simulink model "sim_ukf_est_motor_3para"  (R2020b)
settings: Solver=ode1  StartTime=0.0  StopTime=30  FixedStep=0.01  RelTol=1e-3
undefined symbols (not defined in the file): DiscIntNeverNeededParam
settings Model: Creator=Sarot PC  LastModifiedBy=ONLY-GOD

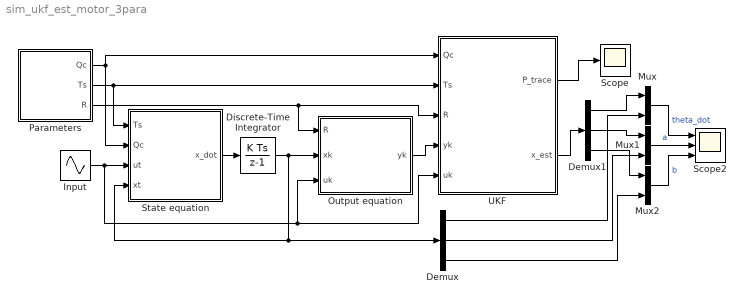
== system sim_ukf_est_motor_3para ==
  Demux : Demux  Outputs=3
  Demux1 : Demux  Outputs=3
  "Discrete-Time Integrator " : DiscreteIntegrator  gainval=1  InitialCondition=[0;20;300]  SampleTime=-1  ICPrevOutput=DiscIntNeverNeededParam  ICPrevScaledInput=DiscIntNeverNeededParam
  Input : Sin  Amplitude=15  SampleTime=0
  Mux : Mux  Inputs=2
  Mux1 : Mux  Inputs=2
  Mux2 : Mux  Inputs=2
  Output equation : MATLAB Function  TreatAsAtomicUnit=on
  Parameters : MATLAB Function  TreatAsAtomicUnit=on
  Scope : Scope
  Scope2 : Scope  NumInputPorts=3
  State equation : MATLAB Function  TreatAsAtomicUnit=on
  UKF : MATLAB Function  TreatAsAtomicUnit=on
  wires:
  Input/1 -> Output equation/3(uk), UKF/5(uk), State equation/3(ut)
  State equation/1(x_dot) -> "Discrete-Time Integrator "/1
  "Discrete-Time Integrator "/1 -> Output equation/2(xk), State equation/4(xt), Demux/1
  Parameters/1(Qc) -> UKF/1(Qc), State equation/2(Qc)
  Parameters/2(Ts) -> State equation/1(Ts), UKF/2(Ts)
  Parameters/3(R) -> UKF/3(R), Output equation/1(R)
  Output equation/1(yk) -> UKF/4(yk)
  UKF/2(x_est) -> Demux1/1
  Demux1/1 -> Mux/1
  Demux/1 -> Mux/2
  Demux1/2 -> Mux1/1
  Demux/2 -> Mux1/2
  Demux1/3 -> Mux2/1
  Demux/3 -> Mux2/2
  UKF/1(P_trace) -> Scope/1
  Mux/1 -> Scope2/1  "theta_dot"
  Mux1/1 -> Scope2/2  "a"
  Mux2/1 -> Scope2/3  "b"

== matlab function sim_ukf_est_motor_3para/Output equation ==
  data: R input; yk output size=[1,1]; xk input; uk input
function yk = fcn(R,xk,uk)

persistent m
m = 1; % number of output or measurement
y_tem = hd(uk,xk) + sqrt(R)*randn(m,1);
yk = y_tem(1:1,1);
end

% Customized function

function y = hd(~,x)
C = [1,0,0];
y = C*x;
end

== matlab function sim_ukf_est_motor_3para/State equation ==
  data: Ts input; Qc input; ut input; x_dot output; xt input
function x_dot = fcn(Ts,Qc,ut,xt)

persistent n
n = 3; % number of state
% Stochastic model
x_dot = fc(ut,xt) + sqrt(Qc)/sqrt(Ts)*randn(n,1);
end

% Deterministic model
function x_dot = fc(u,x)
% theta_ddot = -a*theta_dot + b*u-csign(theta_dot)
% Let x(1)=theta_dot (omega), x(2)=a, x(3)=b, then
% x_dot(1) = -x(1)*x(2) + x(3)*u
% x_dot(2) = 0    (since a is constant)
% x_dot(3) = 0    (since b is constant)
% In compact form
% x_dot = fc(u,x)
x_dot = zeros(3,1);
x_dot(1,1) = -x(1,1)*x(2,1) + x(3,1)*u;
x_dot(2,1) = 0;
x_dot(3,1) = 0;
end

== matlab function sim_ukf_est_motor_3para/Parameters ==
  data: Qc output; Ts output; R output
function [Qc,Ts,R]  = fcn()

Ts = 0.01;
Qc = 1e-6*diag([0.1;0.1;15]);
R = 0.000002;

== matlab function sim_ukf_est_motor_3para/UKF ==
  data: P_trace output; Qc input; x_est output; Ts input; R input; yk input size=[1,1]; uk input
function [P_trace,x_est] = fcn(Qc,Ts,R,yk,uk)

persistent n m xk1 Pk1 wm W lambda nsigma
n = 3; % number of state
m = 1; % number of output

if isempty(xk1)
    xk1= randn(n,1); Pk1 = 1e-1*eye(n);
    nsigma = 2*n+1; k=2;
    alpha=0.5; beta=1;
    lambda=alpha^2*(n+k)-n;
    Wm0=lambda/(n+lambda);
    Wc0=lambda/((n+lambda)+(1-alpha^2+beta));
    Wmi=1/2/(n+lambda);
    Wci=Wmi;
    wm=Wmi*ones(nsigma,1); wm(1)=Wm0;
    W=(eye(nsigma)-wm*ones(1,nsigma))...
     *diag([Wc0 Wci*ones(1,2*n)])...
     *(eye(nsigma)-wm*ones(1,nsigma))';
end

%Measurement Update
%Generate Sigma Points
x = xk1; P = Pk1;
A   = chol(P,'lower');
X   = x*ones(1,nsigma) + ...
        sqrt(n+lambda)*[zeros(n,1) A -A];
Y   = zeros(m,nsigma);
for i=1:nsigma
    Y(:,i)= hd(uk,X(:,i));
end
y   = Y*wm;
Pxy = X*W*Y';
Pyy = Y*W*Y'+R;
K   = Pxy/Pyy;
x   = x + K*(yk-y);
P   = P - K*Pyy*K';

%Time Update
%Generate Sigma Points
A = chol(P,'lower');
X = x*ones(1,nsigma) + ...
        sqrt(n+lambda)*[zeros(n,1) A -A];
Xk1 = zeros(n,nsigma);
for i=1:nsigma
    Xk1(:,i)= fd(uk,X(:,i),Ts);
end
xk1     = Xk1*wm;
Pk1     = Xk1*W*Xk1'+Qc*Ts;
x_est   = xk1(1:3,1);
P_trace = trace(Pk1);
end

function y = hd(~,x)
C = [1,0,0];
y = C*x;
end

% Customizable function fc for various equation
function xk1 = fd(u,x,Ts)

% Continuous function
% function x_dot = fc(u,x)
% theta_ddot = -a*theta_do + b*u
% Let x(1)=theta_dot, x(2)=a, x(3)=b, x(4)=c, then
% x_dot(1) = x(2)
% x_dot(2) = -x(3)*x(2) + x(4)*u
% x_dot(3) = 0    (since a is constant)
% x_dot(4) = 0    (since b is constant)
% In compact form
% x_dot = fc(u,x)
x_dot = zeros(3,1);
x_dot(1,1) = -x(1,1)*x(2,1) + x(3,1)*u;
x_dot(2,1) = 0;
x_dot(3,1) = 0;
% end

% Discretization
xk1 = x + x_dot*Ts;
end
